simulink model "Rayleigh_threepath_demo_2003b"  (R2023b)
settings: Solver=VariableStepDiscrete  StartTime=0.0  StopTime=20.0  RelTol=1e-3  EnableMultiTasking=on
undefined symbols (not defined in the file or in its folder): doppler
libraries: commchan3 x2
settings Model: Creator=morelos_zaragoza  LastModifiedBy=14083
settings SolverCC: AlgebraicLoopSolver=TrustRegion
settings DataIOCC: LimitDataPoints=on  SaveFormat=Array  SignalLoggingSaveFormat=ModelDataLogs  ReturnWorkspaceOutputs=off
settings OptimizationCC: ExpressionDepthLimit=2147483647  LifeSpan=inf
settings DebuggingCC: UnderspecifiedInitializationDetection=Classic  MergeDetectMultiDrivingBlocksExec=none  SolverPrmCheckMsg=warning  FcnCallInpInsideContextMsg=warning  UnconnectedInputMsg=warning  UnconnectedOutputMsg=warning  UnconnectedLineMsg=warning  StateNameClashWarn=warning  SFUnexpectedBacktrackingDiag=warning  SFNoUnconditionalDefaultTransitionDiag=warning  SFExecutionAtInitializationDiag=none  ArithmeticOperatorsInVariantConditions=warning
settings HardwareCC: ProdBitPerPointer=32  ProdBitPerSizeT=32  ProdBitPerPtrDiffT=32  ProdLargestAtomicFloat=None  ProdIntDivRoundTo=Undefined  ProdEndianess=Unspecified  ProdWordSize=32  ProdHWDeviceType=32-bit Generic
settings ModelReferenceCC: EnableRefExpFcnMdlSchedulingChecks=on  PropagateSignalLabelsOutOfModel=off
settings SFSimCC: SimUseLocalCustomCode=off  CustomCodeUndefinedFunction=UseInterfaceOnly
settings RTWCC: RTWUseLocalCustomCode=off  DLArmComputeVersion=19.05
settings CodeAppCC: StateflowObjectComments=on
settings GRTTargetCC: TargetLangStandard=C89/C90 (ANSI)  CombineOutputUpdateFcns=off  GRTInterface=on
settings ConfigComp: CovMetricSettings=dw  CovSaveCumulativeToWorkspaceVar=on  CovSaveSingleToWorkspaceVar=on  CovExternalEMLEnable=off

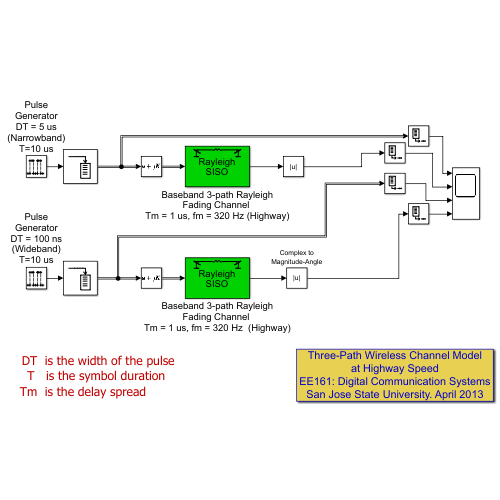
[thumbnail: Simulink's stored preview of the top-level diagram]
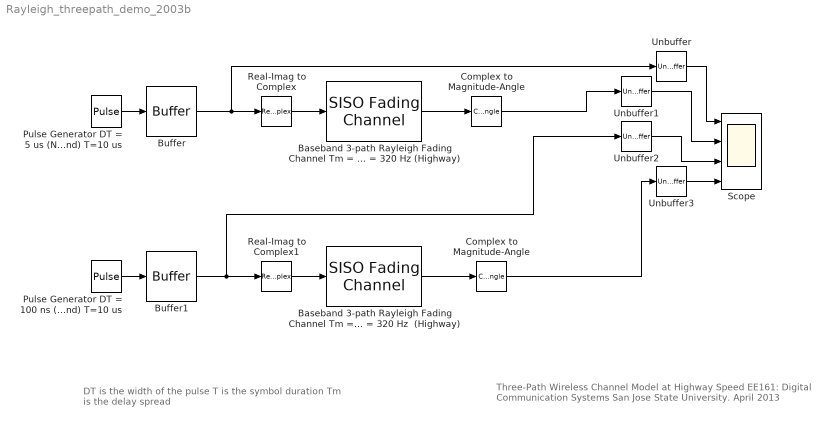
== system Rayleigh_threepath_demo_2003b ==
  note: Three-Path Wireless Channel Model
      | at Highway Speed
      | EE161: Digital Communication Systems
      | San Jose State University. April 2013
  note: DT is the width of the pulse
      | T is the symbol duration
      | Tm is the delay spread
  "Baseband 3-path Rayleigh Fading Channel Tm = 1 us, fm = 320 Hz  (Highway)" : commchan3/SISO Fading Channel  InheritSampleRate=on  SampleRate=1  PathDelays=[0 0.25e-6 1e-6]  AveragePathGains=[0 -1 -2]  NormalizePathGains=on  FadingDistribution=Rayleigh  KFactor=3  DirectPathDopplerShift=0  DirectPathInitialPhase=0  MaximumDopplerShift=320  DopplerSpectrum=doppler('Jakes')  RandomStream=mt19937ar with seed  Seed=43523777  PathGainsOutputPort=off  ChannelFilterDelayOutputPort=off  SimulateUsing=Interpreted execution  Visualization=Off  PathsForDopplerDisplay=1  SamplesToDisplay=25%
  "Baseband 3-path Rayleigh Fading Channel Tm = 1 us, fm = 320 Hz (Highway)" : commchan3/SISO Fading Channel  InheritSampleRate=on  SampleRate=1  PathDelays=[0 0.25e-6 1e-6]  AveragePathGains=[0 -1 -2]  NormalizePathGains=on  FadingDistribution=Rayleigh  KFactor=3  DirectPathDopplerShift=0  DirectPathInitialPhase=0  MaximumDopplerShift=320  DopplerSpectrum=doppler('Jakes')  RandomStream=mt19937ar with seed  Seed=43523777  PathGainsOutputPort=off  ChannelFilterDelayOutputPort=off  SimulateUsing=Interpreted execution  Visualization=Off  PathsForDopplerDisplay=1  SamplesToDisplay=25%
  Buffer : Buffer  N=128
  Buffer1 : Buffer  N=128
  "Complex to Magnitude-Angle " : ComplexToMagnitudeAngle  Output=Magnitude
  Complex to Magnitude-Angle : ComplexToMagnitudeAngle  Output=Magnitude
  Pulse Generator DT = 100 ns (Wideband) T=10 us : DiscretePulseGenerator  Period=1000  PulseWidth=10  SampleTime=1e-8  VectorParams1D=off
  Pulse Generator DT = 5 us (Narrowband) T=10 us : DiscretePulseGenerator  Period=1000  PulseWidth=500  SampleTime=1e-8  VectorParams1D=off
  Real-Imag to Complex : RealImagToComplex  Input=Real
  Real-Imag to Complex1 : RealImagToComplex  Input=Real
  Scope : Scope  NumInputPorts=4
  Unbuffer{,1..3} (4 alike) : Unbuffer
  wires:
  Pulse Generator DT = 5 us (Narrowband) T=10 us/1 -> Buffer/1
  Real-Imag to Complex/1 -> "Baseband 3-path Rayleigh Fading Channel Tm = 1 us, fm = 320 Hz (Highway)"/1
  "Baseband 3-path Rayleigh Fading Channel Tm = 1 us, fm = 320 Hz (Highway)"/1 -> Complex to Magnitude-Angle/1
  Complex to Magnitude-Angle/1 -> Unbuffer1/1
  Pulse Generator DT = 100 ns (Wideband) T=10 us/1 -> Buffer1/1
  Real-Imag to Complex1/1 -> "Baseband 3-path Rayleigh Fading Channel Tm = 1 us, fm = 320 Hz  (Highway)"/1
  "Baseband 3-path Rayleigh Fading Channel Tm = 1 us, fm = 320 Hz  (Highway)"/1 -> "Complex to Magnitude-Angle "/1
  "Complex to Magnitude-Angle "/1 -> Unbuffer3/1
  Buffer/1 -> Real-Imag to Complex/1, Unbuffer/1
  Buffer1/1 -> Real-Imag to Complex1/1, Unbuffer2/1
  Unbuffer/1 -> Scope/1
  Unbuffer1/1 -> Scope/2
  Unbuffer3/1 -> Scope/4
  Unbuffer2/1 -> Scope/3
